simulink model "controller_attitude_yaw"  (R2021a)
settings: configuration reference "Configuration" (kept outside this file)
undefined symbols (not defined in the file): G_Y_OL_DENOM, G_Y_OL_NUM, K_psi, sim_freq
settings Model: DataDictionary=shared_config.sldd  Creator=francois  LastModifiedBy=esl
settings ConfigSetRef: SourceName=Configuration

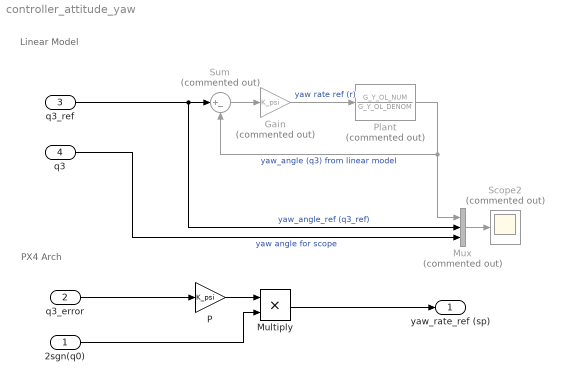
== system controller_attitude_yaw ==
  note: Linear Model
  note: PX4 Arch
  2sgn(q0) : Inport  SampleTime=1/sim_freq
  q3_error : Inport  Port=2  SampleTime=1/sim_freq
  q3_ref : Inport  Port=3
  q3 : Inport  Port=4  SampleTime=1/sim_freq
  Gain : Gain  Commented=on  Gain=K_psi
  Multiply : Product
  Mux : Mux  Commented=on  Inputs=3
  P : Gain  Gain=K_psi
  Plant : TransferFcn  Commented=on  Numerator=G_Y_OL_NUM  Denominator=G_Y_OL_DENOM
  Scope2 : Scope  Commented=on
  Sum : Sum  Commented=on  Inputs=|+-
  yaw_rate_ref (sp) : Outport  VectorParamsAs1DForOutWhenUnconnected=off
  wires:
  q3_ref/1 -> Mux/2, Sum/1  "yaw_angle_ref (q3_ref)"
  Plant/1 -> Mux/1, Sum/2  "yaw_angle (q3) from linear model"
  Sum/1 -> Gain/1
  Gain/1 -> Plant/1  "yaw rate ref (r)"
  P/1 -> Multiply/1
  2sgn(q0)/1 -> Multiply/2
  q3_error/1 -> P/1
  Multiply/1 -> yaw_rate_ref (sp)/1
  q3/1 -> Mux/3  "yaw angle for scope"
  Mux/1 -> Scope2/1
